simulink model "hexacopter"  (R2022a)
settings: Solver=VariableStepAuto  StartTime=0.0  StopTime=10.0  FixedStep=0.01  RelTol=1e-3  EnableMultiTasking=on
InitFcn:
  | params = parameters();
settings Model: Creator=fmina  LastModifiedBy=sebas
settings SolverCC: AlgebraicLoopSolver=TrustRegion
settings DataIOCC: ReturnWorkspaceOutputs=off
settings OptimizationCC: LifeSpan=inf
settings DebuggingCC: UnconnectedInputMsg=warning  UnconnectedOutputMsg=warning  UnconnectedLineMsg=warning  SFUnexpectedBacktrackingDiag=warning  SFNoUnconditionalDefaultTransitionDiag=warning  SFExecutionAtInitializationDiag=none  SFMachineParentedDataDiag=warning  ArithmeticOperatorsInVariantConditions=warning
settings SFSimCC: SimUseLocalCustomCode=off  CustomCodeUndefinedFunction=UseInterfaceOnly
settings RTWCC: RTWUseLocalCustomCode=off  DLArmComputeVersion=19.05
settings CodeAppCC: StateflowObjectComments=on
settings GRTTargetCC: TargetLangStandard=C89/C90 (ANSI)
settings ConfigComp: CovMetricSettings=dw  CovSaveCumulativeToWorkspaceVar=on  CovSaveSingleToWorkspaceVar=on  CovExternalEMLEnable=off

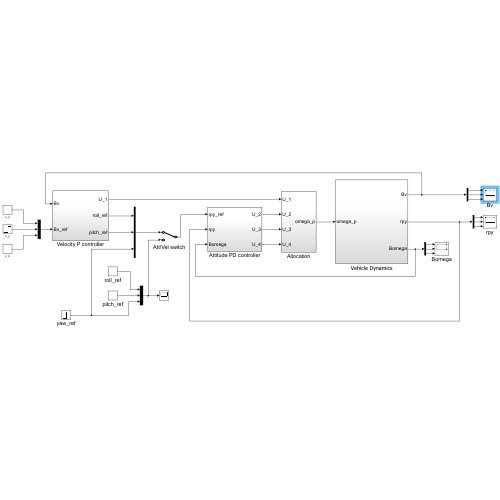
[thumbnail: Simulink's stored preview of the top-level diagram]
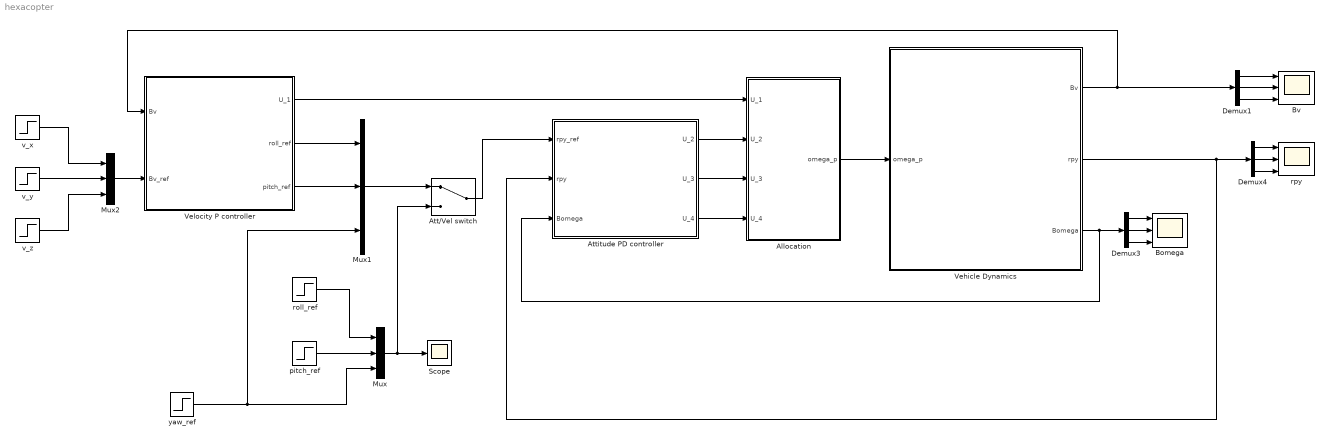
== system hexacopter ==
  Allocation : Subsystem
  Att/Vel switch : ManualSwitch
  Attitude PD controller : Subsystem
  Bomega : Scope  NumInputPorts=3
  Bv : Scope  NumInputPorts=3
  Demux1 : Demux  Outputs=3
  Demux3 : Demux  Outputs=3
  Demux4 : Demux  Outputs=3
  Mux : Mux  Inputs=3
  Mux1 : Mux  Inputs=3
  Mux2 : Mux  Inputs=3
  Scope : Scope
  Vehicle Dynamics : Subsystem
  Velocity P controller : Subsystem
  pitch_ref : Step  Time=3  After=0.25  SampleTime=0
  roll_ref : Step  After=0.24  SampleTime=0
  rpy : Scope  NumInputPorts=3
  v_x : Step  After=0.25  SampleTime=0
  v_y : Step  Time=3  After=0.25  SampleTime=0
  v_z : Step  Time=5  After=0.25  SampleTime=0
  yaw_ref : Step  Time=5  After=0  SampleTime=0
  wires:
  Demux1/2 -> Bv/2
  Demux1/3 -> Bv/3
  Demux1/1 -> Bv/1
  Demux3/2 -> Bomega/2
  Demux3/3 -> Bomega/3
  Demux3/1 -> Bomega/1
  Demux4/1 -> rpy/1
  Demux4/2 -> rpy/2
  Demux4/3 -> rpy/3
  roll_ref/1 -> Mux/1
  pitch_ref/1 -> Mux/2
  yaw_ref/1 -> Mux/3, Mux1/3
  Att/Vel switch/1 -> Attitude PD controller/1(rpy_ref)
  Velocity P controller/3(pitch_ref) -> Mux1/2
  Velocity P controller/2(roll_ref) -> Mux1/1
  Mux/1 -> Scope/1, Att/Vel switch/2
  Mux1/1 -> Att/Vel switch/1
  Mux2/1 -> Velocity P controller/2(Bv_ref)
  v_x/1 -> Mux2/1
  v_y/1 -> Mux2/2
  v_z/1 -> Mux2/3
  Velocity P controller/1(U_1) -> Allocation/1(U_1)
  Attitude PD controller/1(U_2) -> Allocation/2(U_2)
  Attitude PD controller/2(U_3) -> Allocation/3(U_3)
  Attitude PD controller/3(U_4) -> Allocation/4(U_4)
  Vehicle Dynamics/3(Bomega) -> Demux3/1, Attitude PD controller/3("Bomega ")
  Vehicle Dynamics/1(Bv) -> Demux1/1, Velocity P controller/1(Bv)
  Allocation/1(omega_p) -> Vehicle Dynamics/1(omega_p)
  Vehicle Dynamics/2(rpy) -> Demux4/1, Attitude PD controller/2(rpy)

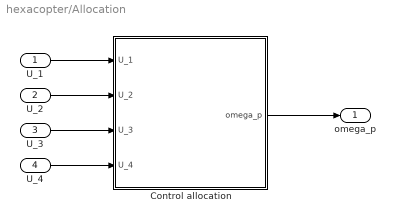
== system hexacopter/Allocation ==
  U_1 : Inport
  U_2 : Inport  Port=2
  U_3 : Inport  Port=3
  U_4 : Inport  Port=4
  Control allocation : MATLAB Function  TreatAsAtomicUnit=on
  omega_p : Outport  PortDimensions=[6,1]
  wires:
  U_1/1 -> Control allocation/1(U_1)
  Control allocation/1(omega_p) -> omega_p/1
  U_4/1 -> Control allocation/4(U_4)
  U_2/1 -> Control allocation/2(U_2)
  U_3/1 -> Control allocation/3(U_3)

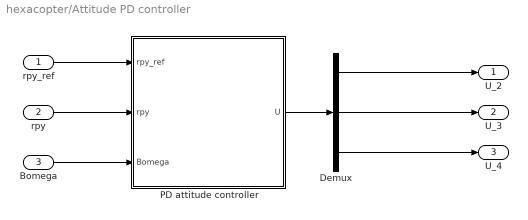
== system hexacopter/Attitude PD controller ==
  rpy_ref : Inport
  rpy : Inport  Port=2
  "Bomega " : Inport  Port=3
  Demux : Demux  Outputs=3
  PD attitude controller : MATLAB Function  TreatAsAtomicUnit=on
  U_2 : Outport
  U_3 : Outport  Port=2
  U_4 : Outport  Port=3
  wires:
  rpy_ref/1 -> PD attitude controller/1(rpy_ref)
  rpy/1 -> PD attitude controller/2(rpy)
  "Bomega "/1 -> PD attitude controller/3(Bomega)
  PD attitude controller/1(U) -> Demux/1
  Demux/1 -> U_2/1
  Demux/2 -> U_3/1
  Demux/3 -> U_4/1

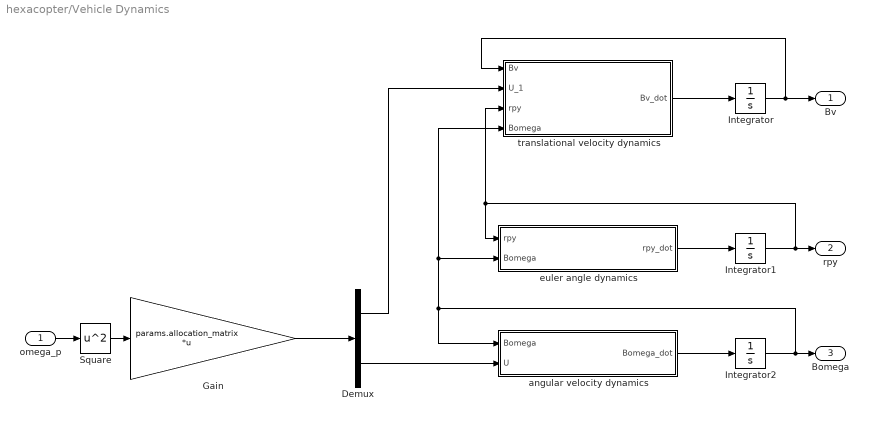
== system hexacopter/Vehicle Dynamics ==
  omega_p : Inport
  Demux : Demux  Outputs=[1 3]
  Gain : Gain  Gain=params.allocation_matrix  Multiplication=Matrix(K*u)
  Integrator : Integrator  InitialCondition=params.Bv_0
  Integrator1 : Integrator  InitialCondition=params.rpy_0
  Integrator2 : Integrator  InitialCondition=[0;0;0]
  Square : Math  Operator=square
  angular velocity dynamics : MATLAB Function  TreatAsAtomicUnit=on
  euler angle dynamics : MATLAB Function  TreatAsAtomicUnit=on
  translational velocity dynamics : MATLAB Function  TreatAsAtomicUnit=on
  Bv : Outport
  rpy : Outport  Port=2
  Bomega : Outport  Port=3
  wires:
  Gain/1 -> Demux/1
  Integrator/1 -> translational velocity dynamics/1(Bv), Bv/1
  Integrator1/1 -> translational velocity dynamics/3(rpy), euler angle dynamics/1(rpy), rpy/1
  Integrator2/1 -> Bomega/1, angular velocity dynamics/1(Bomega), euler angle dynamics/2(Bomega), translational velocity dynamics/4(Bomega)
  Demux/2 -> angular velocity dynamics/2(U)
  angular velocity dynamics/1(Bomega_dot) -> Integrator2/1
  euler angle dynamics/1(rpy_dot) -> Integrator1/1
  translational velocity dynamics/1(Bv_dot) -> Integrator/1
  Demux/1 -> translational velocity dynamics/2(U_1)
  omega_p/1 -> Square/1
  Square/1 -> Gain/1

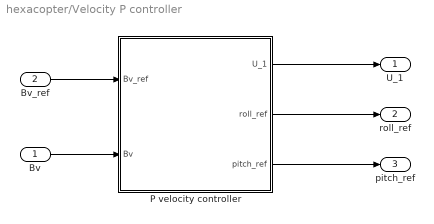
== system hexacopter/Velocity P controller ==
  Bv : Inport
  Bv_ref : Inport  Port=2
  P velocity controller : MATLAB Function  TreatAsAtomicUnit=on
  U_1 : Outport
  roll_ref : Outport  Port=2
  pitch_ref : Outport  Port=3
  wires:
  Bv_ref/1 -> P velocity controller/1(Bv_ref)
  Bv/1 -> P velocity controller/2(Bv)
  P velocity controller/1(U_1) -> U_1/1
  P velocity controller/3(pitch_ref) -> pitch_ref/1
  P velocity controller/2(roll_ref) -> roll_ref/1

== matlab function hexacopter/Vehicle Dynamics/euler angle dynamics ==
  data: rpy input; Bomega input; rpy_dot output
function rpy_dot = rpy_dyn(rpy, Bomega)
params = parameters();
% input
% rpy: current attitude rpy = [roll; pitch; yaw]
% Bomega: current angular velocity expressed in body frame

% output
% rpy_dot: roll, pitch and yaw time derivative

% TODO: compute the roll, pitch and yaw time derivative
rpy_dot = [0; 0; 0];

rpy_dot = Bomega;

end

== matlab function hexacopter/Vehicle Dynamics/angular velocity dynamics ==
  data: Bomega input; U input; Bomega_dot output
function Bomega_dot = Bomega_dyn(Bomega, U)
params = parameters();
% input
% Bomega: current angular velocity expressed in body frame
% U: body torque U = [U_2; U_3; U_4]

% output
% Bomega_dot: angular velocity time derivative expressed in body frame

% TODO: compute the angular velocity time derivative
Bomega_dot = [0; 0; 0];

Bomega_dot = inv(params.J) * U;
end

== matlab function hexacopter/Vehicle Dynamics/translational velocity dynamics ==
  data: Bv input; U_1 input; rpy input; Bv_dot output; Bomega input
function Bv_dot = Bv_dyn(Bv, U_1, rpy, Bomega)
params = parameters();
% input
% Bv: current translational velocity expressed in body frame
% U_1: thrust force
% rpy: current attitude rpy = [roll; pitch; yaw]
% Bomega: current angular velocity expressed in body frame

% output
% Bv_dot: translational velocity time derivative expressed in body frame

% TODO: compute the translational velocity time derivative
Bv_dot = [0; 0; 0];

Bv_dot = [params.g * rpy(2); - params.g * rpy(1); U_1 / params.m - params.g];

end

== matlab function hexacopter/Attitude PD controller/PD attitude controller ==
  data: rpy_ref input; U output; rpy input; Bomega input
function U = PD_att_ctrl(rpy_ref, rpy, Bomega)
params = parameters();
% input
% rpy_ref: reference roll, pitch and yaw angles
% rpy: current roll, pitch and yaw angles;
% Bomega: current angular velocity expressed in body frame

% output
% U: control torques U = [U_2; U_3; U_4]

% TODO: compute the control torques required to track the desired attitude
U = zeros(3,1);

Kp = diag(params.attitude_Kp);
Kd = diag(params.attitude_Kd);

U = Kp * (rpy_ref - rpy) - Kd * Bomega;

== matlab function hexacopter/Velocity P controller/P velocity controller ==
  data: Bv_ref input; U_1 output; Bv input; roll_ref output; pitch_ref output
function [U_1, roll_ref, pitch_ref] = P_vel_ctrl(Bv_ref, Bv)
params = parameters();

% input:
% Bv_ref: velocity reference expressed in body frame
% Bv: current velocity expressed in body frame

% output:
% U_1: thrust force
% roll_ref: desired roll angle
% pitch_ref: desired pitch angle 

% TODO: compute the thrust force, roll and pitch angle required to track
% the desired velocity
U_1 = 0;
roll_ref = 0;
pitch_ref = 0;

m = params.m;
g = params.g;
Kp = params.velocity_Kp;
error = Bv_ref - Bv;

U_1 = Kp(3) * error(3) + m*g;
roll_ref = -Kp(2) * error(2);
pitch_ref = Kp(1) * error(1);

== matlab function hexacopter/Allocation/Control allocation ==
  data: U_1 input; omega_p output; U_2 input; U_3 input; U_4 input
function omega_p = alloc(U_1, U_2, U_3, U_4)
params = parameters();
omega_p_sqr = params.pinv_allocation_matrix*[U_1; U_2; U_3; U_4];

%make sure only positive values are allowed.
omega_p_sqr = max(omega_p_sqr, zeros(6,1));

%actual rotors velocities
omega_p = sqrt(omega_p_sqr);
